simulink model "ejemplo1"  (R2013b)
settings: Solver=ode45  StartTime=0.0  StopTime=10.0  RelTol=1e-3
settings Model: Creator=user  LastModifiedBy=user
settings DataIOCC: SaveFormat=StructureWithTime  SaveState=on

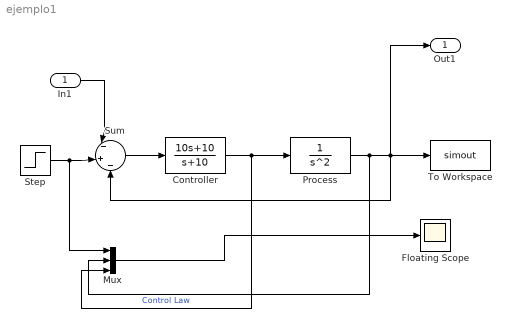
== system ejemplo1 ==
  In1 : Inport
  Controller : TransferFcn  Numerator=[10 10]  Denominator=[1 10]
  Floating Scope : Scope
  Mux : Mux  Inputs=3
  Process : TransferFcn  Denominator=[1 0 0]
  Step : Step  SampleTime=0
  Sum : Sum  Inputs=|-|+|-
  To Workspace : ToWorkspace  VariableName=simout  SampleTime=-1  SaveFormat=Timeseries
  Out1 : Outport
  wires:
  Step/1 -> Mux/1, Sum/2
  In1/1 -> Sum/1
  Sum/1 -> Controller/1
  Controller/1 -> Mux/3, Process/1  "Control Law"
  Process/1 -> Mux/2, Sum/3, Out1/1, To Workspace/1
  Mux/1 -> Floating Scope/1
